simulink model "grid_tied_inverter_mppt"  (R2021a)
settings: Solver=FixedStepAuto  StartTime=0.0  StopTime=18  FixedStep=Tss  RelTol=1e-3
values from neighbouring files (symbols this model uses):
  f = 50    [three_phase_inverter_para.m]
  Lf = ((0.1*V^2)/(2*pi*f*Pmin))    (= 0.00612852634199)    [three_phase_inverter_para.m]
  Rlf = Lf*25    (= 0.15321315855)    [three_phase_inverter_para.m]
  Tss = 10e-6    (= 1e-05)    [three_phase_inverter_para.m]
  V = 380    [three_phase_inverter_para.m]
undefined symbols (not defined in the file or in its folder): sigbuilder_block
libraries: pid_lib x2, spsThreePhaseVIMeasurementLib x2, spsSeriesRLCBranchLib x1, spsPLL3phLib x1, spsPVArrayLib x1, spsPWMGenerator2LevelLib x1, spsPower3phInstantaneousLib x1, spsTHDLib x1, spsThreePhaseSeriesRLCBranchLib x1, spsThreePhaseSourceLib x1, spsUniversalBridgeLib x1, spsabctodq0Lib x1
settings Model: Creator=ACER  LastModifiedBy=ACER

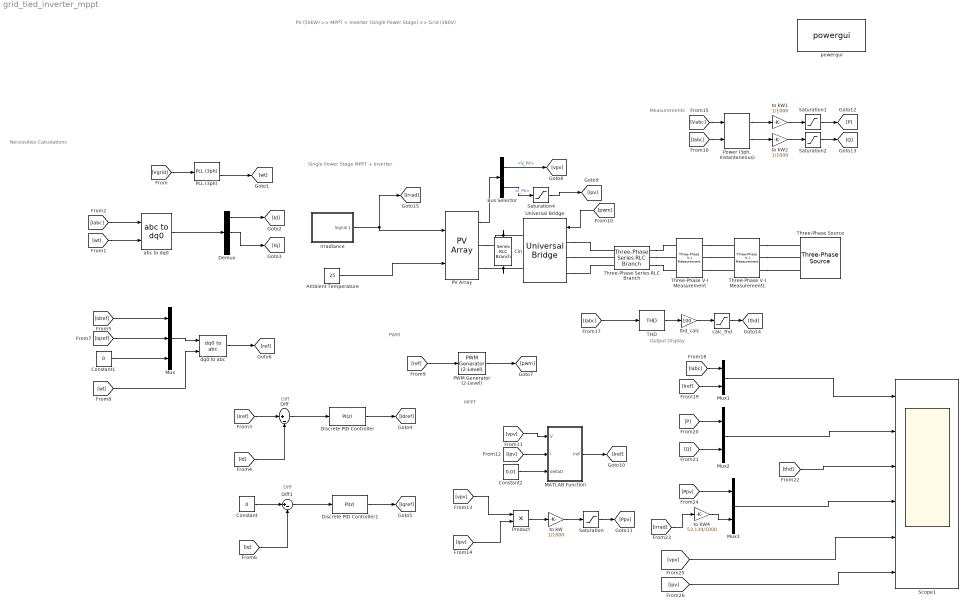
== system grid_tied_inverter_mppt ==
  note: PV (50kW) >> MPPT + Inverter (Single Power Stage) >> Grid (380V)
  note: Measurements
  note: PWM
  note: MPPT
  note: Output Display
  note: Necessities Calculations
  note: Single Power Stage MPPT + Inverter
  note: Diff
  note: Diff
  Ambient Temperature : Constant  Value=25
  Bus Selector : BusSelector  OutputSignals=V_PV,I_PV
  Cin : spsSeriesRLCBranchLib/Series RLC Branch  LConnTagsString=__new0  RConnTagsString=__new0  BranchType=RC  Resistance=1e-3  Inductance=1e-3  SetiL0=off  InitialCurrent=0  Capacitance=100e-6  Setx0=off  InitialVoltage=0  Measurements=None
  Constant : Constant  Value=0
  Constant1 : Constant  Value=0
  Constant2 : Constant  Value=0.01
  Demux : Demux  Outputs=3
  Diff : Sum  Inputs=|+-
  Diff1 : Sum  Inputs=|+-
  Discrete PID Controller : pid_lib/PID Controller  Controller=PI  Form=Parallel  TimeDomain=Discrete-time  UseExternalTs=off  SampleTime=Tss*10  IntegratorMethod=Forward Euler  FilterMethod=Forward Euler  ControllerParametersSource=internal  P=0.005  I=1  D=0  UseFilter=on  N=100  TunerSelectOption=Transfer Function Based (PID Tuner App)  InitialConditionSource=internal  InitialConditionForIntegrator=0  InitialConditionForFilter=0  DifferentiatorICPrevScaledInput=0  ExternalReset=none  TrackingMode=off  Kt=1  LimitOutput=on  SatLimitsSource=internal  UpperSaturationLimit=1.2  LowerSaturationLimit=0  LinearizeAsGain=off  AntiWindupMode=none  Kb=1  POutMin=[]  POutMax=[]  IOutMin=[]  IOutMax=[]  DOutMin=[]  DOutMax=[]  NOutMin=[]  NOutMax=[]  SumOutMin=[]  SumOutMax=[]  SaturationOutMin=[]  SaturationOutMax=[]  PParamMin=[]  PParamMax=[]  IParamMin=[]  IParamMax=[]  DParamMin=[]  DParamMax=[]  NParamMin=[]  NParamMax=[]  KbParamMin=[]  KbParamMax=[]  KtParamMin=[]  KtParamMax=[]  KbOutMin=[]  KbOutMax=[]  KtOutMin=[]  KtOutMax=[]  IntegratorOutMin=[]  IntegratorOutMax=[]  FilterOutMin=[]  FilterOutMax=[]  SumI1OutMin=[]  SumI1OutMax=[]  SumI2OutMin=[]  SumI2OutMax=[]  SumI3OutMin=[]  SumI3OutMax=[]  SumI4OutMin=[]  SumI4OutMax=[]  SumDOutMin=[]  SumDOutMax=[]  DifferentiatorOutMin=[]  DifferentiatorOutMax=[]  FilterDiffOutCoefMin=[]  FilterDiffOutCoefMax=[]  ReciprocalOutMin=[]  ReciprocalOutMax=[]  SumDenOutMin=[]  SumDenOutMax=[]  SumNumOutMin=[]  SumNumOutMax=[]  DivideOutMin=[]  DivideOutMax=[]  UdiffTsProdOutMin=[]  UdiffTsProdOutMax=[]  NTsProdOutMin=[]  NTsProdOutMax=[]  UintegralTsProdOutMin=[]  UintegralTsProdOutMax=[]  UngainTsProdOutMin=[]  UngainTsProdOutMax=[]  IntegratorContinuousStateAttributes=''  IntegratorStateMustResolveToSignalObject=off  IntegratorRTWStateStorageClass=Auto  FilterContinuousStateAttributes=''  FilterStateMustResolveToSignalObject=off  FilterRTWStateStorageClass=Auto  ParallelPVariant=InternalParameters  IdealPVariant=Disabled  IVariant=InternalParameters  DVariant=Disabled  IntegratorVariant=Discrete  SatVariant=Enabled  AWVariant=Passthrough  PCopyVariant=Disabled  TRVariant=Disabled  FdbkBlocksVariant=Forward  IdealPFdbkVariant=Disabled  SatFdbkVariant=Disabled  DerivativeFilterVariant=Disabled  NVariant=Disabled  NCopyVariant=Disabled_SignalSpec  FilterICVariant=Disabled  IntegratorICVariant=InternalICs  ExternalResetVariant=Disabled  TRSumVariant=Passthrough  SumFdbkVariant=Disabled  SumVariant=Sum_PI  TsampFilterVariant=InternalTs  TsampNgainVariant=Passthrough  TsampIntegralVariant=Passthrough  ExternalSaturationOutDataTypeStr=Inherit: Same as second input
  Discrete PID Controller1 : pid_lib/PID Controller  Controller=PI  Form=Parallel  TimeDomain=Discrete-time  UseExternalTs=off  SampleTime=Tss*10  IntegratorMethod=Forward Euler  FilterMethod=Forward Euler  ControllerParametersSource=internal  P=0.01  I=1  D=0  UseFilter=on  N=100  TunerSelectOption=Transfer Function Based (PID Tuner App)  InitialConditionSource=internal  InitialConditionForIntegrator=0  InitialConditionForFilter=0  DifferentiatorICPrevScaledInput=0  ExternalReset=none  TrackingMode=off  Kt=1  LimitOutput=on  SatLimitsSource=internal  UpperSaturationLimit=1.1  LowerSaturationLimit=-1.1  LinearizeAsGain=off  AntiWindupMode=none  Kb=1  POutMin=[]  POutMax=[]  IOutMin=[]  IOutMax=[]  DOutMin=[]  DOutMax=[]  NOutMin=[]  NOutMax=[]  SumOutMin=[]  SumOutMax=[]  SaturationOutMin=[]  SaturationOutMax=[]  PParamMin=[]  PParamMax=[]  IParamMin=[]  IParamMax=[]  DParamMin=[]  DParamMax=[]  NParamMin=[]  NParamMax=[]  KbParamMin=[]  KbParamMax=[]  KtParamMin=[]  KtParamMax=[]  KbOutMin=[]  KbOutMax=[]  KtOutMin=[]  KtOutMax=[]  IntegratorOutMin=[]  IntegratorOutMax=[]  FilterOutMin=[]  FilterOutMax=[]  SumI1OutMin=[]  SumI1OutMax=[]  SumI2OutMin=[]  SumI2OutMax=[]  SumI3OutMin=[]  SumI3OutMax=[]  SumI4OutMin=[]  SumI4OutMax=[]  SumDOutMin=[]  SumDOutMax=[]  DifferentiatorOutMin=[]  DifferentiatorOutMax=[]  FilterDiffOutCoefMin=[]  FilterDiffOutCoefMax=[]  ReciprocalOutMin=[]  ReciprocalOutMax=[]  SumDenOutMin=[]  SumDenOutMax=[]  SumNumOutMin=[]  SumNumOutMax=[]  DivideOutMin=[]  DivideOutMax=[]  UdiffTsProdOutMin=[]  UdiffTsProdOutMax=[]  NTsProdOutMin=[]  NTsProdOutMax=[]  UintegralTsProdOutMin=[]  UintegralTsProdOutMax=[]  UngainTsProdOutMin=[]  UngainTsProdOutMax=[]  IntegratorContinuousStateAttributes=''  IntegratorStateMustResolveToSignalObject=off  IntegratorRTWStateStorageClass=Auto  FilterContinuousStateAttributes=''  FilterStateMustResolveToSignalObject=off  FilterRTWStateStorageClass=Auto  ParallelPVariant=InternalParameters  IdealPVariant=Disabled  IVariant=InternalParameters  DVariant=Disabled  IntegratorVariant=Discrete  SatVariant=Enabled  AWVariant=Passthrough  PCopyVariant=Disabled  TRVariant=Disabled  FdbkBlocksVariant=Forward  IdealPFdbkVariant=Disabled  SatFdbkVariant=Disabled  DerivativeFilterVariant=Disabled  NVariant=Disabled  NCopyVariant=Disabled_SignalSpec  FilterICVariant=Disabled  IntegratorICVariant=InternalICs  ExternalResetVariant=Disabled  TRSumVariant=Passthrough  SumFdbkVariant=Disabled  SumVariant=Sum_PI  TsampFilterVariant=InternalTs  TsampNgainVariant=Passthrough  TsampIntegralVariant=Passthrough  ExternalSaturationOutDataTypeStr=Inherit: Same as second input
  Irradiance : Subsystem  Tag=STV Subsys  LoadFcn=sigbuilder_block('load');  StartFcn=sigbuilder_block('start');  StopFcn=sigbuilder_block('stop');  ClipboardFcn=sigbuilder_block('clipboard');  mask(Sigbuilder block){tuvar=[0:10]}
      mask help: Simulink:masks:SigbuilderBlock_MD
      mask init:
      | if ~strcmp(get_param(bdroot(gcbh),'SimulationStatus'),'stopped') tuvar = sigbuilder_block('maskInit'); end
      settings: CopyFcn=sigbuilder_block('copy');  DeleteFcn=sigbuilder_block('delete');  ModelCloseFcn=sigbuilder_block('modelClose');  PreSaveFcn=sigbuilder_block('preSave');  PauseFcn=sigbuilder_block('pause');  ContinueFcn=sigbuilder_block('continue');  NameChangeFcn=sigbuilder_block('namechange');  OpenFcn=sigbuilder_block('open',[220.2 153.6 550.8 361.2 ]);  CloseFcn=sigbuilder_block('close');
      mask Display: plot(0, 0, 100, 100,[2, 2, 32, 32, 2], [68, 8, 8, 68, 68],[32, 2], [38, 38], [32, 19, 2],[53, 60, 44], [32, 17, 17, 2],[16, 16, 31, 31]);txt = getActiveGroup(gcbh);text(2, 100, txt,'verticalAlignment', 'top');
  MATLAB Function : MATLAB Function  TreatAsAtomicUnit=on
  Mux : Mux  Inputs=3
  Mux1 : Mux  Inputs=2
  Mux2 : Mux  Inputs=2
  Mux3 : Mux  Inputs=2
  PLL (3ph) : spsPLL3phLib/PLL (3ph)  Fmin=45  Par_Init=[0, 50]  ParK=[180, 3200, 1]  TcD=1e-4  MaxRateChangeFreq=12  FilterCutOffFreq=25  Ts=Tss  AGC=on
  PV Array : spsPVArrayLib/PV Array  Npar=11  Nser=21  PlotType=array @ 25 deg.C & specified irradiances  S_vec="[ 1000  ]"  Temp_C_vec="[ 45 25  ]"  ModuleName=SunPower SPR-230E-WHT-D  PlotWhenSelected=off  Pm=230.04  Ncell=72  Voc=48.2  Isc=6.05  Vm=40.5  Im=5.68  beta_Voc_pc=-0.31  alpha_Isc_pc=0.016  beta_Voc=-0.14942  alpha_Isc=0.000968  IL=6.0553  I0=2.9343e-11  nI=1.0009  Rsh=396.8073  Rs=0.34627  RobustModel=off  RobustCellTemperature=313.3991  BAL=on  Tc=1e-6  Tfilter=5e-5
  PWM Generator (2-Level) : spsPWMGenerator2LevelLib/PWM Generator (2-Level)  ModulatorType=Three-phase bridge (6 pulses)  ModulatorMode=Unsynchronized  Fc=fsw  Pc=90  nF=27  MinMax="[ -1  1 ]"  SamplingTechnique=Natural  ModulatingSignals=off  m=0.8  Freq=60  Phase=0  Ts=Tss  ShowCarrierOutport=off
  "Power (3ph, Instantaneous)" : spsPower3phInstantaneousLib/Power (3ph, Instantaneous)
  Product : Product
  Saturation : Saturate  UpperLimit=60  LowerLimit=0
  Saturation1 : Saturate  UpperLimit=60  LowerLimit=0
  Saturation2 : Saturate
  Saturation4 : Saturate  UpperLimit=200  LowerLimit=0
  Scope1 : Scope  NumInputPorts=6
  THD : spsTHDLib/THD  Freq=50  Ts=Tss
      settings: SourceProductBaseCode=PS
  Three-Phase Series RLC Branch : spsThreePhaseSeriesRLCBranchLib/Three-Phase Series RLC Branch  LConnTagsString=A|B|C  RConnTagsString=A|B|C  BranchType=RL  Resistance=Rlf  Inductance=Lf  Capacitance=1e-6  Measurements=None
  Three-Phase V-I Measurement : spsThreePhaseVIMeasurementLib/Three-Phase V-I Measurement  VoltageMeasurement=phase-to-ground  SetLabelV=on  LabelV=Vabc  Vpu=off  VpuLL=off  CurrentMeasurement=yes  SetLabelI=on  LabelI=Iabc  Ipu=off  Pbase=100e6  Vbase=500e3  OutputType=Complex  PhasorSimulation=off  PSBequivalent=0
  Three-Phase V-I Measurement1 : spsThreePhaseVIMeasurementLib/Three-Phase V-I Measurement  VoltageMeasurement=phase-to-ground  SetLabelV=on  LabelV=Vgrid  Vpu=off  VpuLL=off  CurrentMeasurement=no  SetLabelI=off  LabelI=Iabc  Ipu=off  Pbase=100e6  Vbase=500e3  OutputType=Complex  PhasorSimulation=off  PSBequivalent=0
  Three-Phase Source : spsThreePhaseSourceLib/Three-Phase Source  InternalConnection=Yg  VoltagePhases=off  Voltage=V  PhaseAngle=0  Voltage_phases=[25e3 25e3 25e3]/sqrt(3)  PhaseAngles_phases=[0 -120 +120]  Frequency=f  NonIdealSource=on  SpecifyImpedance=on  Resistance=0.8929  Inductance=16.58e-3  ShortCircuitLevel=100e6  BaseVoltage=V  XRratio=7  BusType=swing  Pref=10e3  Qref=0  Prefabc=[10e3, 10e3, 10e3]  Qrefabc=[0, 0, 0]  Qmin=-inf  Qmax=inf
  Universal Bridge : spsUniversalBridgeLib/Universal Bridge  Arms=3  SnubberResistance=1e5  SnubberCapacitance=inf  Device=IGBT / Diodes  Ron=1e-3  Lon=0  ForwardVoltages="[  0  0  ]"  ForwardVoltage=0  GTOparameters=[ 10e-6 , 20e-6 ]  IGBTparameters=[ 1e-6 , 2e-6 ]  Measurements=None  Measurements_2=None  converterType=Rectifier
  abc to dq0 : spsabctodq0Lib/abc to dq0  Alignment=90 degrees behind phase A axis
  calc_thd : Saturate  UpperLimit=15  LowerLimit=0
  dq0 to abc : spsdq0toabcLib/dq0 to abc  Alignment=90 degrees behind phase A axis
  powergui : spspowerguiLib/powergui  Priority=1  SimulationMode=Discrete  SampleTime=Tss  frequency=60  Iterations=50  frequencyindice=0  Pbase=100e6  ErrMax=1e-4  UnitsV=kV  UnitsW=MW  buscounter=0  FunctionMessages=off  echomessages=off  EnableUseOfTLC=off  CurrentSourceSwitches=off  DisableSnubberDevices=off  DisableRonSwitches=off  DisableVfSwitches=off  DisplayEquations=off  AutomaticDiscreteSolvers=off  SolverType=Tustin/Backward Euler (TBE)  Interpol=off  ExternalGateDelay=off  methode=off  Ts=100  x0status=blocks  SPID=on  SwTol=0  HookPort=off  NonlinearTolerance=1e-4  nMaxIteration=100  ContinueOnMaxIteration=off  RestoreLinks=warning  ResistiveCurrentMeasurement=off  Frange=[0:2:500]  Ylog=off  Xlog=on  ShowGrid=off  save=off  variable=ZData  structure=0  ZoomFFT=off  StartTime=0.0  cycles=1  DisplayStyle=1  fundamental=60  FreqAxis=off  MaxFrequency=1000  frequencyindicesteady=1  RmsSteady=1  display=off
  thd_calc : Gain  Gain=100
  to kW : Gain  Gain=1/1000
  to kW1 : Gain  Gain=1/1000
  to kW2 : Gain  Gain=1/1000
  to kW4 : Gain  Gain=53.139/1000
  wires:
  [Vgrid] -> PLL (3ph)/1
  PLL (3ph)/2 -> [wt]
  [Iabc] -> abc to dq0/1
  [wt] -> abc to dq0/2
  [Iref] -> Diff/1
  [Id] -> Diff/2
  Diff/1 -> Discrete PID Controller/1
  Discrete PID Controller/1 -> [Idref]
  Diff1/1 -> Discrete PID Controller1/1
  [Iq] -> Diff1/2
  Discrete PID Controller1/1 -> [Iqref]
  Constant/1 -> Diff1/1
  [Iqref] -> Mux/2
  [Idref] -> Mux/1
  Mux/1 -> dq0 to abc/1
  [wt] -> dq0 to abc/2
  Constant1/1 -> Mux/3
  dq0 to abc/1 -> [ref]
  [ref] -> PWM Generator (2-Level)/1
  PWM Generator (2-Level)/1 -> [pwm]
  [pwm] -> Universal Bridge/1
  Irradiance/1(Signal 1) -> [irrad], PV Array/1
  Ambient Temperature/1 -> PV Array/2
  PV Array/1 -> Bus Selector/1
  Bus Selector/1 -> [vpv]  "<V_PV>"
  [vpv] -> MATLAB Function/1(V)
  [ipv] -> MATLAB Function/2(I)
  Constant2/1 -> MATLAB Function/3(deltaD)
  MATLAB Function/1(Iref) -> [Iref]
  [vpv] -> Product/1
  [ipv] -> Product/2
  Product/1 -> to kW/1
  to kW/1 -> Saturation/1
  Saturation/1 -> [Ppv]
  [Vabc] -> "Power (3ph, Instantaneous)"/1
  [Iabc] -> "Power (3ph, Instantaneous)"/2
  "Power (3ph, Instantaneous)"/1 -> to kW1/1
  "Power (3ph, Instantaneous)"/2 -> to kW2/1
  to kW1/1 -> Saturation1/1
  to kW2/1 -> Saturation2/1
  Saturation2/1 -> [Q]
  Saturation1/1 -> [P]
  THD/1 -> thd_calc/1
  thd_calc/1 -> calc_thd/1
  calc_thd/1 -> [thd]
  Mux1/1 -> Scope1/1
  [Iabc] -> Mux1/1
  [Iref] -> Mux1/2
  [P] -> Mux2/1
  Mux2/1 -> Scope1/2
  [Q] -> Mux2/2
  [thd] -> Scope1/3
  [irrad] -> to kW4/1
  [Ppv] -> Mux3/1
  to kW4/1 -> Mux3/2
  Mux3/1 -> Scope1/4
  [vpv] -> Scope1/5
  [ipv] -> Scope1/6
  Bus Selector/2 -> Saturation4/1  "<I_PV>"
  Saturation4/1 -> [ipv]
  Demux/1 -> [Id]
  Demux/2 -> [Iq]
  abc to dq0/1 -> Demux/1
  [Iabc] -> THD/1
  connections:
  Universal Bridge/LConn1 -- Three-Phase Series RLC Branch/LConn1
  Universal Bridge/LConn2 -- Three-Phase Series RLC Branch/LConn2
  Universal Bridge/LConn3 -- Three-Phase Series RLC Branch/LConn3
  Three-Phase Series RLC Branch/RConn1 -- Three-Phase V-I Measurement/LConn1
  Three-Phase Series RLC Branch/RConn2 -- Three-Phase V-I Measurement/LConn2
  Three-Phase Series RLC Branch/RConn3 -- Three-Phase V-I Measurement/LConn3
  Three-Phase V-I Measurement/RConn1 -- Three-Phase V-I Measurement1/LConn1
  Three-Phase V-I Measurement/RConn2 -- Three-Phase V-I Measurement1/LConn2
  Three-Phase V-I Measurement/RConn3 -- Three-Phase V-I Measurement1/LConn3
  Three-Phase V-I Measurement1/RConn1 -- Three-Phase Source/RConn1
  Three-Phase V-I Measurement1/RConn2 -- Three-Phase Source/RConn2
  Three-Phase V-I Measurement1/RConn3 -- Three-Phase Source/RConn3
  PV Array/RConn1 -- Universal Bridge/RConn1 -- Cin/LConn1
  PV Array/RConn2 -- Universal Bridge/RConn2 -- Cin/RConn1

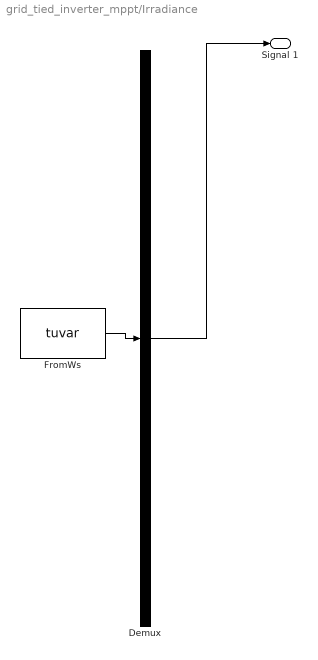
== system grid_tied_inverter_mppt/Irradiance ==
  Demux : Demux  Tag=STV Demux  Outputs=1
      settings: DisplayOption=none
  FromWs : FromWorkspace  Tag=STV FromWs  VariableName=tuvar
      SigBuilderData=|
      | common.afterFinalStr = 'Extrapolate'
      | common.sampleTime = 0
      | dataSet.timeRange = [0 18]
      | dataSet.name = 'Group 1'
      | sbobj.Groups.Name = 'Group 1'
      | sbobj.Groups.Signals.Name = 'Signal 1'
      | sbobj.Groups.Signals.XData = [0 0.0187304890739 0.0374609781478 0.0561914672216 0.0749219562955 0.0936524453694 0.112382934443 0.131113423517 0.149843912591 0.168574401665 0.187304890739 0.206035379813 ... (962 elements, 1x962)]
      | sbobj.Groups.Signals.YData = [2.37993 2.37993 2.37993 2.37993 2.37993 2.37993 2.37993 2.37993 2.37993 2.37992 2.37992 2.37992 ... (962 elements, 1x962)]
      | sbobj.Groups.TimeRange = [0 18]
  Signal 1 : Outport  Tag=STV Outport
  wires:
  FromWs/1 -> Demux/1
  Demux/1 -> Signal 1/1

== matlab function grid_tied_inverter_mppt/MATLAB Function ==
  data: V input; Iref output; I input; deltaD input
function Iref = MPPT(V,I,deltaD)

Iref_init = 0.1;
I_min = 0;
I_max = 150;

persistent Vold  Pold Iref_old;

if isempty(Vold)
    Vold = 0;
    
    Pold = 0;
    
    Iref_old =Iref_init;
    
end

P = V*I;

dV = V - Vold;
dP = P - Pold;

Iref =  Iref_old;

if dP ~=0 && V > 400
    
    if dP < 0 
        if dV < 0 
            
            Iref = Iref_old - deltaD; %shall include in blog why deltaD is subtracted here
            
        else
            Iref = Iref_old + deltaD;
            
        end
    else
        
        if dV < 0
            
            Iref = Iref_old + deltaD;
            
        else
            
            Iref = Iref_old - deltaD;
            
        end
    end
end

if Iref >= I_max
    
    Iref = I_max;
end

if Iref < I_min
    
    Iref = I_min;
    
end

Iref_old = Iref;

Vold = V;
Pold = P;
